simulink model "Hybrid"  (R2018b)
settings: Solver=VariableStepAuto  StartTime=0.0  StopTime=10.0  RelTol=1e-3
settings Model: Creator=yizha  LastModifiedBy=yizha

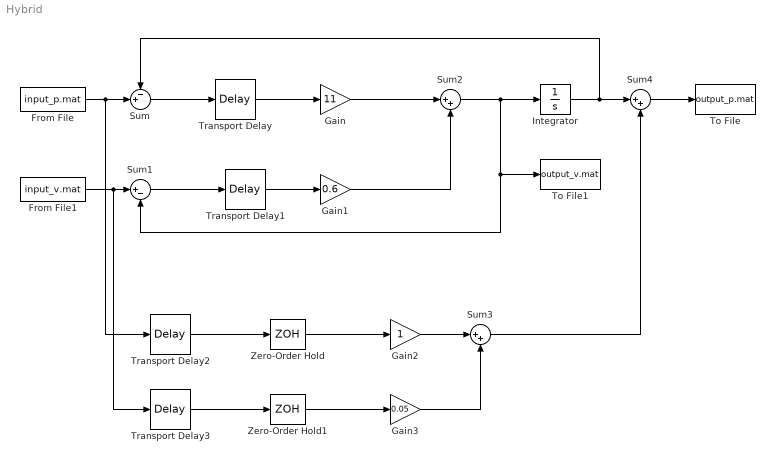
== system Hybrid ==
  From File : FromFile  FileName=input_p.mat  SampleTime=0
  From File1 : FromFile  FileName=input_v.mat  SampleTime=0
  Gain : Gain  Gain=11
  Gain1 : Gain  Gain=0.6
  Gain2 : Gain
  Gain3 : Gain  Gain=0.05
  Integrator : Integrator
  Sum : Sum  Inputs=-+|
  Sum1 : Sum  Inputs=|+-
  Sum2 : Sum  Inputs=|++
  Sum3 : Sum  Inputs=|++
  Sum4 : Sum  Inputs=|++
  To File : ToFile  Filename=output_p.mat
  To File1 : ToFile  Filename=output_v.mat
  Transport Delay{,1..3} (4 alike) : TransportDelay  DelayTime=0.1
  Zero-Order Hold : ZeroOrderHold  SampleTime=0.1
  Zero-Order Hold1 : ZeroOrderHold  SampleTime=0.1
  wires:
  Sum2/1 -> Integrator/1, To File1/1, Sum1/2
  Transport Delay1/1 -> Gain1/1
  From File/1 -> Transport Delay2/1, Sum/2
  Sum1/1 -> Transport Delay1/1
  Integrator/1 -> Sum4/1, Sum/1
  Transport Delay/1 -> Gain/1
  Gain/1 -> Sum2/1
  From File1/1 -> Transport Delay3/1, Sum1/1
  Gain1/1 -> Sum2/2
  Sum/1 -> Transport Delay/1
  Transport Delay2/1 -> Zero-Order Hold/1
  Gain3/1 -> Sum3/2
  Zero-Order Hold/1 -> Gain2/1
  Transport Delay3/1 -> Zero-Order Hold1/1
  Zero-Order Hold1/1 -> Gain3/1
  Gain2/1 -> Sum3/1
  Sum4/1 -> To File/1
  Sum3/1 -> Sum4/2
